simulink model "adaptive_wiener_filter"  (R2020b)
settings: Solver=FixedStepDiscrete  StartTime=0.0  StopTime=stopTime  FixedStep=2.0833333333333333e-05  RelTol=1e-3
values from neighbouring files (symbols this model uses):
  mp = sm_init_avalon_signals(mp)    [sm_callback_init.m]
settings Model: Creator=Ross  LastModifiedBy=conno
settings SolverCC: AutoInsertRateTranBlk=on
settings DataIOCC: SaveOutput=off  SaveTime=off  ReturnWorkspaceOutputs=off
settings OptimizationCC: BlockReduction=off  ConditionallyExecuteInputs=off  DefaultParameterBehavior=Inlined
settings DebuggingCC: SignalInfNanChecking=error  SignalRangeChecking=warning  ReadBeforeWriteMsg=DisableAll  WriteAfterWriteMsg=DisableAll  WriteAfterReadMsg=DisableAll  AlgebraicLoopMsg=error  MultiTaskDSMMsg=none  SingleTaskRateTransMsg=error  ParameterUnderflowMsg=warning  UnderSpecifiedDataTypeMsg=error  PregeneratedLibrarySubsystemCodeDiagnostic=none  ArithmeticOperatorsInVariantConditions=warning
settings HardwareCC: ProdBitPerPointer=32  ProdBitPerSizeT=32  ProdBitPerPtrDiffT=32  ProdLargestAtomicFloat=None  ProdIntDivRoundTo=Undefined  ProdEndianess=Unspecified  ProdWordSize=32  ProdHWDeviceType=ASIC/FPGA->ASIC/FPGA  TargetBitPerPointer=64  TargetBitPerSizeT=64  TargetBitPerPtrDiffT=64  TargetLongLongMode=on  TargetIntDivRoundTo=Zero  TargetEndianess=LittleEndian  TargetWordSize=64  TargetHWDeviceType=Custom Processor->MATLAB Host Computer  ProdEqTarget=off
settings ModelReferenceCC: UpdateModelReferenceTargets=IfOutOfDate
settings SFSimCC: SFSimEcho=off  SimUseLocalCustomCode=off  CustomCodeUndefinedFunction=UseInterfaceOnly
settings RTWCC: RTWUseLocalCustomCode=off

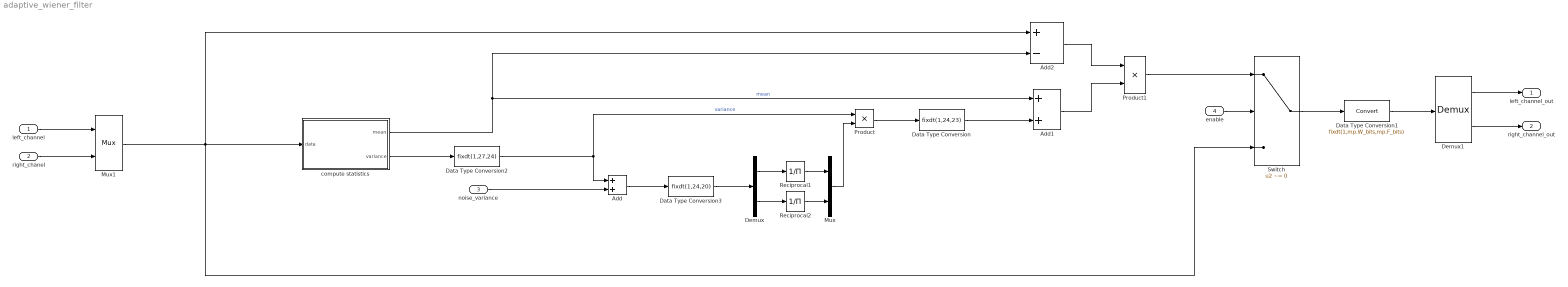
== system adaptive_wiener_filter ==
  left_channel : Inport  OutDataTypeStr=fixdt(1,24,23)  PortDimensions=1  SampleTime=[2.0833333333333333e-05,0]
  right_chanel : Inport  Port=2  OutDataTypeStr=fixdt(1,24,23)  PortDimensions=1  SampleTime=[2.0833333333333333e-05,0]
  noise_variance : Inport  Port=3  OutDataTypeStr=fixdt(0,16,15)  PortDimensions=1  SampleTime=[2.0833333333333333e-05,0]
  enable : Inport  Port=4  OutDataTypeStr=boolean  PortDimensions=1  SampleTime=[2.0833333333333333e-05,0]
  Add : Sum
  Add1 : Sum
  Add2 : Sum  Inputs=+-
  Data Type Conversion : DataTypeConversion  OutDataTypeStr=fixdt(1,24,23)
  Data Type Conversion1 : DataTypeConversion  OutDataTypeStr=fixdt(1,mp.W_bits,mp.F_bits)
  Data Type Conversion2 : DataTypeConversion  OutDataTypeStr=fixdt(1,27,24)
  Data Type Conversion3 : DataTypeConversion  OutDataTypeStr=fixdt(1,24,20)
  Demux : Demux  Outputs=2
  Demux1 : Demux  Outputs=2
      settings: DisplayOption=none
  Mux : Mux  Inputs=2
  Mux1 : Mux  Inputs=2
  Product : Product
  Product1 : Product
  Reciprocal1 : Product  Inputs=/  RndMeth=Zero  SaturateOnIntegerOverflow=on
  Reciprocal2 : Product  Inputs=/  RndMeth=Zero  SaturateOnIntegerOverflow=on
  Switch : Switch  Criteria=u2 ~= 0
  compute statistics : Subsystem
  left_channel_out : Outport  OutDataTypeStr=fixdt(1,24,23)  PortDimensions=1  SampleTime=[2.0833333333333333e-05,0]
  right_channel_out : Outport  Port=2  OutDataTypeStr=fixdt(1,24,23)  PortDimensions=1  SampleTime=[2.0833333333333333e-05,0]
  wires:
  compute statistics/1(mean) -> Add1/1, Add2/2  "mean"
  Data Type Conversion/1 -> Add1/2
  Product/1 -> Data Type Conversion/1
  Data Type Conversion2/1 -> Product/1, Add/1  "variance"
  compute statistics/2(variance) -> Data Type Conversion2/1
  Add2/1 -> Product1/1
  Add1/1 -> Product1/2
  Product1/1 -> Switch/1
  Demux/1 -> Reciprocal1/1
  Demux/2 -> Reciprocal2/1
  Reciprocal2/1 -> Mux/2
  Reciprocal1/1 -> Mux/1
  enable/1 -> Switch/2
  noise_variance/1 -> Add/2
  Add/1 -> Data Type Conversion3/1
  Data Type Conversion3/1 -> Demux/1
  Mux/1 -> Product/2
  right_chanel/1 -> Mux1/2
  Mux1/1 -> compute statistics/1(data), Add2/1, Switch/3
  left_channel/1 -> Mux1/1
  Switch/1 -> Data Type Conversion1/1
  Data Type Conversion1/1 -> Demux1/1
  Demux1/1 -> left_channel_out/1
  Demux1/2 -> right_channel_out/1

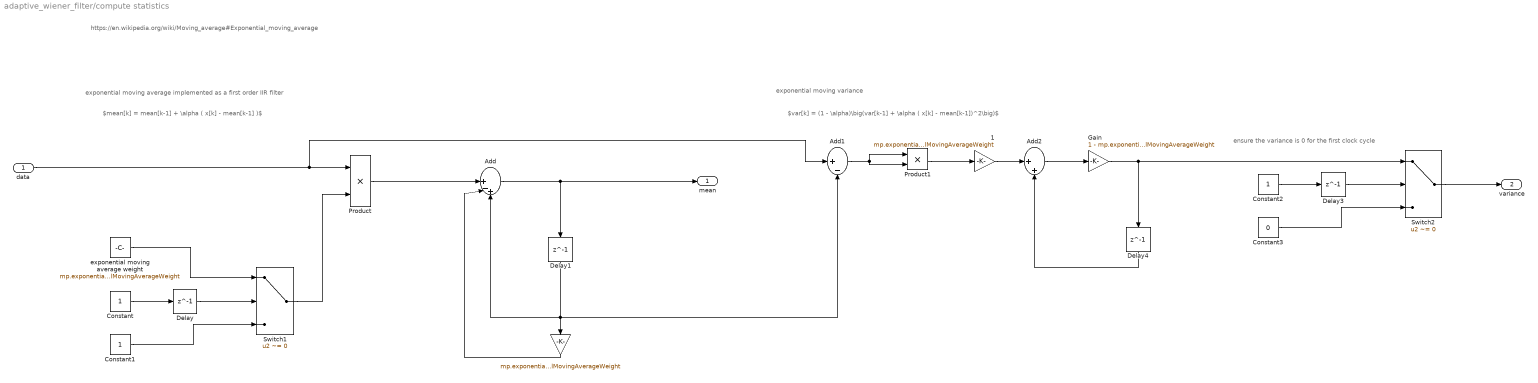
== system adaptive_wiener_filter/compute statistics ==
  note: $var[k] = (1 - \alpha)\big(var[k-1] + \alpha ( x[k] - mean[k-1])^2\big)$
  note: exponential moving average implemented as a first order IIR filter
  note: exponential moving variance
  note: $mean[k] = mean[k-1] + \alpha ( x[k] - mean[k-1] )$
  note: https://en.wikipedia.org/wiki/Moving_average#Exponential_moving_average
  note: ensure the variance is 0 for the first clock cycle
  data : Inport
  " " : Gain  Gain=mp.exponentialMovingAverageWeight  ParamDataTypeStr=Inherit: Inherit from 'Gain'  OutDataTypeStr=Inherit: Inherit via back propagation
  " 1" : Gain  Gain=mp.exponentialMovingAverageWeight  ParamDataTypeStr=Inherit: Inherit from 'Gain'  OutDataTypeStr=Inherit: Same as input
  Add : Sum  Inputs=||+-+  InputSameDT=on  OutDataTypeStr=Inherit: Same as first input
  Add1 : Sum  Inputs=|+-  InputSameDT=on  OutDataTypeStr=Inherit: Same as first input
  Add2 : Sum  Inputs=|++  InputSameDT=on
  Constant : Constant  OutDataTypeStr=boolean  SampleTime=-1
  Constant1 : Constant  OutDataTypeStr=Inherit: Inherit via back propagation  SampleTime=-1
  Constant2 : Constant  OutDataTypeStr=boolean  SampleTime=-1
  Constant3 : Constant  Value=0  OutDataTypeStr=Inherit: Inherit via back propagation  SampleTime=-1
  Delay{,1,3..4} (4 alike) : Delay  DelayLength=1  InitialCondition=0
  Gain : Gain  Gain=1 - mp.exponentialMovingAverageWeight  ParamDataTypeStr=Inherit: Inherit from 'Gain'  OutDataTypeStr=Inherit: Same as input
  Product : Product  OutDataTypeStr=Inherit: Same as first input
  Product1 : Product  OutMin=-2  OutMax=2  OutDataTypeStr=fixdt(1,50)
  Switch1 : Switch  Criteria=u2 ~= 0  InputSameDT=on
  Switch2 : Switch  Criteria=u2 ~= 0  InputSameDT=on
  exponential moving average weight : Constant  Value=mp.exponentialMovingAverageWeight  SampleTime=-1
  mean : Outport  InitialOutput=0
  variance : Outport  Port=2  InitialOutput=0
  wires:
  Delay4/1 -> Add2/2
  Gain/1 -> Delay4/1, Switch2/1
  Delay1/1 -> Add/3, " "/1, Add1/2
  Add/1 -> Delay1/1, mean/1
  " 1"/1 -> Add2/1
  Switch2/1 -> variance/1
  Constant3/1 -> Switch2/3
  Delay3/1 -> Switch2/2
  Constant2/1 -> Delay3/1
  data/1 -> Product/1, Add1/1
  Product1/1 -> " 1"/1
  exponential moving average weight/1 -> Switch1/1
  Product/1 -> Add/1
  Delay/1 -> Switch1/2
  Constant1/1 -> Switch1/3
  " "/1 -> Add/2
  Add1/1 -> Product1/1, Product1/2
  Add2/1 -> Gain/1
  Switch1/1 -> Product/2
  Constant/1 -> Delay/1
